simulink model "Kalman_Filter_Example"  (R2019b)
settings: Solver=VariableStepAuto  StartTime=0.0  StopTime=10.0  RelTol=1e-3
undefined symbols (not defined in the file or in its folder): Discrete, Time
libraries: simulink x1, ctrlSharedLib x1
settings Model: Creator=crbon  LastModifiedBy=Chris

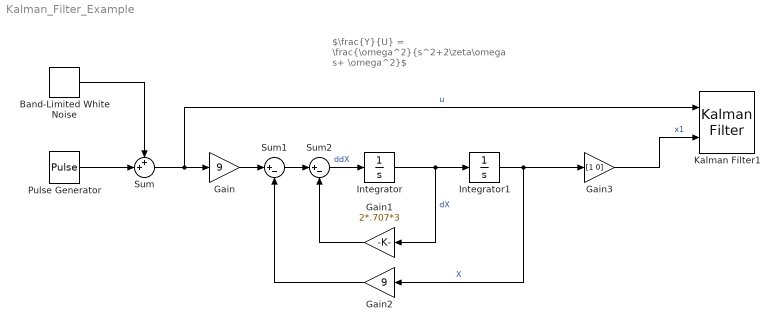
== system Kalman_Filter_Example ==
  note: $\frac{Y}{U} = \frac{\omega^2}{s^2+2\zeta\omega s+ \omega^2}$
  Band-Limited White Noise : simulink/Sources/Band-Limited White Noise  Cov=[0.1]  Ts=0.1  seed=[23341]
  Gain : Gain  Gain=9
  Gain1 : Gain  Gain=2*.707*3
  Gain2 : Gain  Gain=9
  Gain3 : Gain  Gain=[1 0]
  Integrator : Integrator
  Integrator1 : Integrator
  Kalman Filter1 : ctrlSharedLib/Kalman Filter  TimeDomain=Discrete-Time  UseCurrentEstimator=on  ModelSource=Individual A, B, C, D matrices  ModelSourceVariable=ss(0.95,1,1,0,1)  A=[1 1/200; -9/200 -2*.707*3/200]  B=0  C=[1 0]  D=0  NumberOfStates=1  NumberOfInputs=1  NumberOfOutputs=1  InitialEstimateSource=Dialog  X0=0  P0=10  UseK=off  UseGH=off  NumberOfProcessNoiseInputs=1  G=1  TimeInvariantG=on  H=0  TimeInvariantH=on  Q=0.05  TimeInvariantQ=on  R=1  TimeInvariantR=on  N=0  TimeInvariantN=on  AddInputPort=on  AddEnablePort=off  OutputEstimatedY=off  OutputP=off  Ts=-1
      settings: SourceProductBaseCode=CT
  Pulse Generator : DiscretePulseGenerator  PulseType=Time based  Period=10  PulseWidth=5
  Sum : Sum  Inputs=++|
  Sum1 : Sum  Inputs=|+-
  Sum2 : Sum  Inputs=|+-
  wires:
  Pulse Generator/1 -> Sum/2
  Band-Limited White Noise/1 -> Sum/1
  Sum/1 -> Kalman Filter1/1, Gain/1  "u"
  Gain/1 -> Sum1/1
  Sum1/1 -> Sum2/1
  Sum2/1 -> Integrator/1  "ddX"
  Gain1/1 -> Sum2/2
  Integrator/1 -> Integrator1/1, Gain1/1  "dX"
  Gain2/1 -> Sum1/2
  Integrator1/1 -> Gain2/1, Gain3/1  "X"
  Gain3/1 -> Kalman Filter1/2  "x1"
